simulink model "dof_ex_1_sim"  (R2025b)
settings: Solver=VariableStepAuto  StartTime=0.0  StopTime=Tend  RelTol=1e-3
values from neighbouring files (symbols this model uses):
  delta1 = 0    [dof.m]    (also in dof_ex_1.m = 1)
  delta2 = 1    [dof.m]
  rho = 0    [dof.m]    (also in dof_ex_1.m)
  Ts = 2e-3    (= 0.002)    [dof.m]    (also in dof_ex_1.m = 0.005)
libraries: cstblocks x2, simulink x2
settings Model: Creator=davidecovolo  LastModifiedBy=davidecovolo

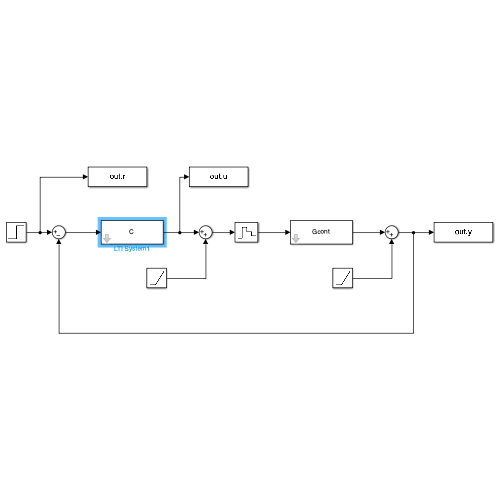
[thumbnail: Simulink's stored preview of the top-level diagram]
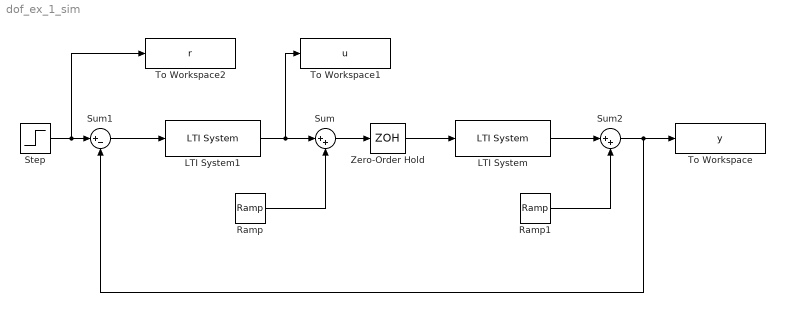
== system dof_ex_1_sim ==
  LTI System : cstblocks/LTI System  sys=Gcont  IC=[]  PadeOrder=0
  LTI System1 : cstblocks/LTI System  sys=C  IC=[]  PadeOrder=0
  Ramp : simulink/Sources/Ramp  slope=delta1  start=0  InitialOutput=0
  Ramp1 : simulink/Sources/Ramp  slope=delta2  start=0  InitialOutput=0
  Step : Step  Time=0  After=rho  SampleTime=0
  Sum : Sum  Inputs=|++
  Sum1 : Sum  Inputs=|+-
  Sum2 : Sum  Inputs=|++
  To Workspace : ToWorkspace  VariableName=y  SaveFormat=Timeseries  SampleTime=-1
  To Workspace1 : ToWorkspace  VariableName=u  SaveFormat=Timeseries  SampleTime=-1
  To Workspace2 : ToWorkspace  VariableName=r  SaveFormat=Timeseries  SampleTime=-1
  Zero-Order Hold : ZeroOrderHold  SampleTime=Ts
  wires:
  Zero-Order Hold/1 -> LTI System/1
  Sum/1 -> Zero-Order Hold/1
  LTI System1/1 -> To Workspace1/1, Sum/1
  Ramp/1 -> Sum/2
  Sum1/1 -> LTI System1/1
  Step/1 -> To Workspace2/1, Sum1/1
  Ramp1/1 -> Sum2/2
  LTI System/1 -> Sum2/1
  Sum2/1 -> Sum1/2, To Workspace/1
